simulink model "phan_tich_he_thong_ss"  (R2025a)
settings: Solver=VariableStepAuto  StartTime=0.0  StopTime=20  RelTol=1e-3
undefined symbols (not defined in the file or in its folder): sys
settings Model: SimulationMode=accelerator  Creator=datng  LastModifiedBy=datng

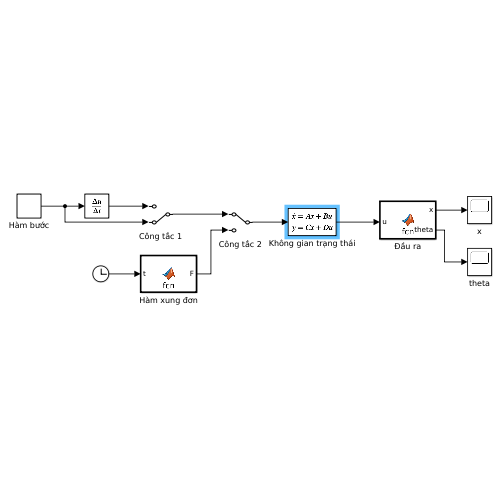
[thumbnail: Simulink's stored preview of the top-level diagram]
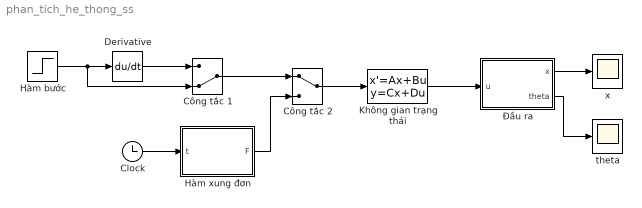
== system phan_tich_he_thong_ss ==
  Clock : Clock
  Công tắc 1 : ManualSwitch  CurrentSetting=0
  Công tắc 2 : ManualSwitch
  Derivative : Derivative
  Hàm bước : Step  Time=0  SampleTime=0
  Hàm xung đơn : MATLAB Function  TreatAsAtomicUnit=on
  Không gian trạng thái : StateSpace  A=sys.A  B=sys.B  C=sys.C  D=sys.D  InitialCondition=0  ContinuousStateAttributes={'x', 'dot_x', 'theta', 'dot_theta'}
  theta : Scope
      settings: ActiveDisplayYMinimum=-0.0052273873149966624  ActiveDisplayYMaximum=0.047046485834969967
  x : Scope
      settings: ActiveDisplayYMinimum=-7.3371176612404  ActiveDisplayYMaximum=66.034058951163615
  Đầu ra : MATLAB Function  TreatAsAtomicUnit=on
  wires:
  Hàm xung đơn/1(F) -> Công tắc 2/2
  Clock/1 -> Hàm xung đơn/1(t)
  Hàm bước/1 -> Công tắc 1/2, Derivative/1
  Derivative/1 -> Công tắc 1/1
  Công tắc 1/1 -> Công tắc 2/1
  Công tắc 2/1 -> Không gian trạng thái/1
  Không gian trạng thái/1 -> Đầu ra/1(u)
  Đầu ra/1(x) -> x/1
  Đầu ra/2(theta) -> theta/1

== matlab function phan_tich_he_thong_ss/Hàm xung đơn ==
  data: t input; F output
function F = fcn(t)
    if t >= 0 && t <= 5
        F = 5;
    else
        F = 0;
    end
end

== matlab function phan_tich_he_thong_ss/Đầu ra ==
  data: u input; x output; theta output
function [x, theta] = fcn(u)
    x = u(1, :);
    theta = u(2, :);
end
